simulink library "inp"  (R2021b)
settings: Solver=VariableStepAuto  StartTime=0.0  StopTime=10.0  RelTol=1e-3
undefined symbols (not defined in the file): C_TASK_5MS_S, FALSE, KINP_AcoreReadyToSlp_flg_ovrdflg, KINP_AcoreReadyToSlp_flg_ovrdval, KINP_AllowMovThd_OTA_enum_ovrdflg, KINP_AllowMovThd_OTA_enum_ovrdval, KINP_APSAngleTarget_Deg_ovrdflg, KINP_APSAngleTarget_Deg_ovrdval, KINP_APSDecReq_mps2_ovrdflg, KINP_APSDecReq_mps2_ovrdval, KINP_APSDecReqA_flg_ovrdflg, KINP_APSDecReqA_flg_ovrdval, KINP_APSDFLL_cm_ovrdflg, KINP_APSDFLL_cm_ovrdval, KINP_APSDFLR_cm_ovrdflg, KINP_APSDFLR_cm_ovrdval, KINP_APSDRLL_cm_ovrdflg, KINP_APSDRLL_cm_ovrdval, KINP_APSDRLR_cm_ovrdflg, KINP_APSDRLR_cm_ovrdval, KINP_APSExitCondition_enum_ovrdflg, KINP_APSExitCondition_enum_ovrdval, KINP_APSHWVer_enum_ovrdflg, KINP_APSHWVer_enum_ovrdval, KINP_APSProgressPCT_pct_ovrdflg, KINP_APSProgressPCT_pct_ovrdval, KINP_APSPwrReq_enum_ovrdflg, KINP_APSPwrReq_enum_ovrdval, KINP_APSReq_enum_ovrdflg, KINP_APSReq_enum_ovrdval, KINP_APSRQDisplay_enum_ovrdflg, KINP_APSRQDisplay_enum_ovrdval, KINP_APSRqEPASCtrl_flg_ovrdflg, KINP_APSRqEPASCtrl_flg_ovrdval, KINP_APSShiftPosnReq_enum_ovrdval, KINP_APSShiftPosnReq_enum_ovrflg, KINP_APSSpeedCMD_kph_ovrdval, KINP_APSSpeedCMD_kph_ovrflg, KINP_APSStaSystem_enum_ovrdflg, KINP_APSStaSystem_enum_ovrdval, KINP_APSSWVer_enum_ovrdflg, KINP_APSSWVer_enum_ovrdval, KINP_APSVMCReqA_flg_ovrdval, KINP_APSVMCReqA_flg_ovrflg, KINP_APSVRqEPASCtrl_flg_ovrdflg, KINP_APSVRqEPASCtrl_flg_ovrdval, KINP_AuxBattVolmV_mV_ovrdflg, KINP_AuxBattVolmV_mV_ovrdval, KINP_CAASSta_enum_ovrdflg, KINP_CAASSta_enum_ovrdval, KINP_CAASVMCReqA_flg_ovrdval, KINP_CAASVMCReqA_flg_ovrflg, KINP_CAN1BusOff_flg_ovrdflg, KINP_CAN1BusOff_flg_ovrdval, KINP_CAN2BusOff_flg_ovrdflg, KINP_CAN2BusOff_flg_ovrdval, KINP_CAN3BusOff_flg_ovrdflg, KINP_CAN3BusOff_flg_ovrdval, KINP_CAN4BusOff_flg_ovrdflg, KINP_CAN4BusOff_flg_ovrdval ... (+152)
libraries: FVT_lib x1035, hcu_lib x1
(part 18 of 33)

== system inp/INP/CAN3/SignalCheck/BMS1 ==
  BHAL_outputs : Inport
  inp_CanValid_bus : Inport  Port=2
  BMS1CSErr : FVT_lib/inp/can_signal_template  SystemSampleTime=-1  VariantActivationTime=update diagram  Latency=0  AutoFrameSizeCalculation=off
      link override defval: Value=KINP_BMS1CSErr_flg_defval
      link override ovrdflg: Value=KINP_BMS1CSErr_flg_ovrdflg
      link override ovrdval: Value=KINP_BMS1CSErr_flg_ovrdval
  BMS1RCErr : FVT_lib/inp/can_signal_template  SystemSampleTime=-1  VariantActivationTime=update diagram  Latency=0  AutoFrameSizeCalculation=off
      link override defval: Value=KINP_BMS1RCErr_flg_defval
      link override ovrdflg: Value=KINP_BMS1RCErr_flg_ovrdflg
      link override ovrdval: Value=KINP_BMS1RCErr_flg_ovrdval
  BMSChckSum1 : FVT_lib/inp/can_signal_template  SystemSampleTime=-1  VariantActivationTime=update diagram  Latency=0  AutoFrameSizeCalculation=off
      link override defval: Value=KINP_BMSChckSum1_enum_defval
      link override ovrdflg: Value=KINP_BMSChckSum1_enum_ovrdflg
      link override ovrdval: Value=KINP_BMSChckSum1_enum_ovrdval
  BMSRolCnct1 : FVT_lib/inp/can_signal_template  SystemSampleTime=-1  VariantActivationTime=update diagram  Latency=0  AutoFrameSizeCalculation=off
      link override defval: Value=KINP_BMSRolCnct1_enum_defval
      link override ovrdflg: Value=KINP_BMSRolCnct1_enum_ovrdflg
      link override ovrdval: Value=KINP_BMSRolCnct1_enum_ovrdval
  HVBPwrAvailChrg : FVT_lib/inp/can_signal_template  SystemSampleTime=-1  VariantActivationTime=update diagram  Latency=0  AutoFrameSizeCalculation=off
      link override defval: Value=KINP_HVBPwrAvailChrg_kW_defval
      link override ovrdflg: Value=KINP_HVBPwrAvailChrg_kW_ovrdflg
      link override ovrdval: Value=KINP_HVBPwrAvailChrg_kW_ovrdval
  HVBPwrAvailChrg30 : FVT_lib/inp/can_signal_template  SystemSampleTime=-1  VariantActivationTime=update diagram  Latency=0  AutoFrameSizeCalculation=off
      link override defval: Value=KINP_HVBPwrAvailChrg30_kW_defval
      link override ovrdflg: Value=KINP_HVBPwrAvailChrg30_kW_ovrdflg
      link override ovrdval: Value=KINP_HVBPwrAvailChrg30_kW_ovrdval
  HVBPwrAvailChrg60 : FVT_lib/inp/can_signal_template  SystemSampleTime=-1  VariantActivationTime=update diagram  Latency=0  AutoFrameSizeCalculation=off
      link override defval: Value=KINP_HVBPwrAvailChrg60_kW_defval
      link override ovrdflg: Value=KINP_HVBPwrAvailChrg60_kW_ovrdflg
      link override ovrdval: Value=KINP_HVBPwrAvailChrg60_kW_ovrdval
  HVBPwrAvailDchrg : FVT_lib/inp/can_signal_template  SystemSampleTime=-1  VariantActivationTime=update diagram  Latency=0  AutoFrameSizeCalculation=off
      link override defval: Value=KINP_HVBPwrAvailDchrg_kW_defval
      link override ovrdflg: Value=KINP_HVBPwrAvailDchrg_kW_ovrdflg
      link override ovrdval: Value=KINP_HVBPwrAvailDchrg_kW_ovrdval
  HVBPwrAvailDchrg30 : FVT_lib/inp/can_signal_template  SystemSampleTime=-1  VariantActivationTime=update diagram  Latency=0  AutoFrameSizeCalculation=off
      link override defval: Value=KINP_HVBPwrAvailDchrg30_kW_defval
      link override ovrdflg: Value=KINP_HVBPwrAvailDchrg30_kW_ovrdflg
      link override ovrdval: Value=KINP_HVBPwrAvailDchrg30_kW_ovrdval
  HVBPwrAvailDchrg60 : FVT_lib/inp/can_signal_template  SystemSampleTime=-1  VariantActivationTime=update diagram  Latency=0  AutoFrameSizeCalculation=off
      link override defval: Value=KINP_HVBPwrAvailDchrg60_kW_defval
      link override ovrdflg: Value=KINP_HVBPwrAvailDchrg60_kW_ovrdflg
      link override ovrdval: Value=KINP_HVBPwrAvailDchrg60_kW_ovrdval
  HVBattCurr : FVT_lib/inp/can_signal_template  SystemSampleTime=-1  VariantActivationTime=update diagram  Latency=0  AutoFrameSizeCalculation=off
      link override defval: Value=KINP_HVBattCurr_A_defval
      link override ovrdflg: Value=KINP_HVBattCurr_A_ovrdflg
      link override ovrdval: Value=KINP_HVBattCurr_A_ovrdval
  HVBattVolt : FVT_lib/inp/can_signal_template  SystemSampleTime=-1  VariantActivationTime=update diagram  Latency=0  AutoFrameSizeCalculation=off
      link override defval: Value=KINP_HVBattVolt_V_defval
      link override ovrdflg: Value=KINP_HVBattVolt_V_ovrdflg
      link override ovrdval: Value=KINP_HVBattVolt_V_ovrdval
  Terminator_{1..12} (12 alike) : Terminator
  True_VHAL_BMS1CSErr_flg : Constant  Value=TRUE  OutDataTypeStr=boolean
  True_VHAL_BMS1RCErr_flg : Constant  Value=TRUE  OutDataTypeStr=boolean
  True_VHAL_BMSChckSum1_enum : Constant  Value=TRUE  OutDataTypeStr=boolean
  True_VHAL_BMSRolCnct1_enum : Constant  Value=TRUE  OutDataTypeStr=boolean
  True_VHAL_HVBPwrAvailChrg30_kW : Constant  Value=TRUE  OutDataTypeStr=boolean
  True_VHAL_HVBPwrAvailChrg60_kW : Constant  Value=TRUE  OutDataTypeStr=boolean
  True_VHAL_HVBPwrAvailChrg_kW : Constant  Value=TRUE  OutDataTypeStr=boolean
  True_VHAL_HVBPwrAvailDchrg30_kW : Constant  Value=TRUE  OutDataTypeStr=boolean
  True_VHAL_HVBPwrAvailDchrg60_kW : Constant  Value=TRUE  OutDataTypeStr=boolean
  True_VHAL_HVBPwrAvailDchrg_kW : Constant  Value=TRUE  OutDataTypeStr=boolean
  True_VHAL_HVBattCurr_A : Constant  Value=TRUE  OutDataTypeStr=boolean
  True_VHAL_HVBattVolt_V : Constant  Value=TRUE  OutDataTypeStr=boolean
  slr1_{1..12} (12 alike) : BusSelector  OutputSignals=VINP_CANMsgValidBMS1_flg
  slr_VHAL_BMS1CSErr_flg : BusSelector  OutputSignals=VHAL_BMS1CSErr_flg
  slr_VHAL_BMS1RCErr_flg : BusSelector  OutputSignals=VHAL_BMS1RCErr_flg
  slr_VHAL_BMSChckSum1_enum : BusSelector  OutputSignals=VHAL_BMSChckSum1_enum
  slr_VHAL_BMSRolCnct1_enum : BusSelector  OutputSignals=VHAL_BMSRolCnct1_enum
  slr_VHAL_HVBPwrAvailChrg30_kW : BusSelector  OutputSignals=VHAL_HVBPwrAvailChrg30_kW
  slr_VHAL_HVBPwrAvailChrg60_kW : BusSelector  OutputSignals=VHAL_HVBPwrAvailChrg60_kW
  slr_VHAL_HVBPwrAvailChrg_kW : BusSelector  OutputSignals=VHAL_HVBPwrAvailChrg_kW
  slr_VHAL_HVBPwrAvailDchrg30_kW : BusSelector  OutputSignals=VHAL_HVBPwrAvailDchrg30_kW
  slr_VHAL_HVBPwrAvailDchrg60_kW : BusSelector  OutputSignals=VHAL_HVBPwrAvailDchrg60_kW
  slr_VHAL_HVBPwrAvailDchrg_kW : BusSelector  OutputSignals=VHAL_HVBPwrAvailDchrg_kW
  slr_VHAL_HVBattCurr_A : BusSelector  OutputSignals=VHAL_HVBattCurr_A
  slr_VHAL_HVBattVolt_V : BusSelector  OutputSignals=VHAL_HVBattVolt_V
  VINP_BMS1CSErr_flg : Outport
  VINP_BMS1RCErr_flg : Outport  Port=2
  VINP_BMSChckSum1_enum : Outport  Port=3
  VINP_BMSRolCnct1_enum : Outport  Port=4
  VINP_HVBPwrAvailChrg_kW : Outport  Port=5
  VINP_HVBPwrAvailChrg30_kW : Outport  Port=6
  VINP_HVBPwrAvailChrg60_kW : Outport  Port=7
  VINP_HVBPwrAvailDchrg_kW : Outport  Port=8
  VINP_HVBPwrAvailDchrg30_kW : Outport  Port=9
  VINP_HVBPwrAvailDchrg60_kW : Outport  Port=10
  VINP_HVBattCurr_A : Outport  Port=11
  VINP_HVBattVolt_V : Outport  Port=12
  wires:
  BHAL_outputs/1 -> [BHAL_outputs]
  inp_CanValid_bus/1 -> [inp_CanValid_bus]
  [BHAL_outputs] -> slr_VHAL_BMS1CSErr_flg/1
  slr_VHAL_BMS1CSErr_flg/1 -> BMS1CSErr/1  "<VHAL_BMS1CSErr_flg>"
  True_VHAL_BMS1CSErr_flg/1 -> BMS1CSErr/2
  [inp_CanValid_bus] -> slr1_1/1
  slr1_1/1 -> BMS1CSErr/3  "<VINP_CANMsgValidBMS1_flg>"
  BMS1CSErr/1 -> VINP_BMS1CSErr_flg/1  "VINP_BMS1CSErr_flg"
  BMS1CSErr/2 -> Terminator_1/1
  [BHAL_outputs] -> slr_VHAL_BMS1RCErr_flg/1
  slr_VHAL_BMS1RCErr_flg/1 -> BMS1RCErr/1  "<VHAL_BMS1RCErr_flg>"
  True_VHAL_BMS1RCErr_flg/1 -> BMS1RCErr/2
  [inp_CanValid_bus] -> slr1_2/1
  slr1_2/1 -> BMS1RCErr/3  "<VINP_CANMsgValidBMS1_flg>"
  BMS1RCErr/1 -> VINP_BMS1RCErr_flg/1  "VINP_BMS1RCErr_flg"
  BMS1RCErr/2 -> Terminator_2/1
  [BHAL_outputs] -> slr_VHAL_BMSChckSum1_enum/1
  slr_VHAL_BMSChckSum1_enum/1 -> BMSChckSum1/1  "<VHAL_BMSChckSum1_enum>"
  True_VHAL_BMSChckSum1_enum/1 -> BMSChckSum1/2
  [inp_CanValid_bus] -> slr1_3/1
  slr1_3/1 -> BMSChckSum1/3  "<VINP_CANMsgValidBMS1_flg>"
  BMSChckSum1/1 -> VINP_BMSChckSum1_enum/1  "VINP_BMSChckSum1_enum"
  BMSChckSum1/2 -> Terminator_3/1
  [BHAL_outputs] -> slr_VHAL_BMSRolCnct1_enum/1
  slr_VHAL_BMSRolCnct1_enum/1 -> BMSRolCnct1/1  "<VHAL_BMSRolCnct1_enum>"
  True_VHAL_BMSRolCnct1_enum/1 -> BMSRolCnct1/2
  [inp_CanValid_bus] -> slr1_4/1
  slr1_4/1 -> BMSRolCnct1/3  "<VINP_CANMsgValidBMS1_flg>"
  BMSRolCnct1/1 -> VINP_BMSRolCnct1_enum/1  "VINP_BMSRolCnct1_enum"
  BMSRolCnct1/2 -> Terminator_4/1
  [BHAL_outputs] -> slr_VHAL_HVBPwrAvailChrg_kW/1
  slr_VHAL_HVBPwrAvailChrg_kW/1 -> HVBPwrAvailChrg/1  "<VHAL_HVBPwrAvailChrg_kW>"
  True_VHAL_HVBPwrAvailChrg_kW/1 -> HVBPwrAvailChrg/2
  [inp_CanValid_bus] -> slr1_5/1
  slr1_5/1 -> HVBPwrAvailChrg/3  "<VINP_CANMsgValidBMS1_flg>"
  HVBPwrAvailChrg/1 -> VINP_HVBPwrAvailChrg_kW/1  "VINP_HVBPwrAvailChrg_kW"
  HVBPwrAvailChrg/2 -> Terminator_5/1
  [BHAL_outputs] -> slr_VHAL_HVBPwrAvailChrg30_kW/1
  slr_VHAL_HVBPwrAvailChrg30_kW/1 -> HVBPwrAvailChrg30/1  "<VHAL_HVBPwrAvailChrg30_kW>"
  True_VHAL_HVBPwrAvailChrg30_kW/1 -> HVBPwrAvailChrg30/2
  [inp_CanValid_bus] -> slr1_6/1
  slr1_6/1 -> HVBPwrAvailChrg30/3  "<VINP_CANMsgValidBMS1_flg>"
  HVBPwrAvailChrg30/1 -> VINP_HVBPwrAvailChrg30_kW/1  "VINP_HVBPwrAvailChrg30_kW"
  HVBPwrAvailChrg30/2 -> Terminator_6/1
  [BHAL_outputs] -> slr_VHAL_HVBPwrAvailChrg60_kW/1
  slr_VHAL_HVBPwrAvailChrg60_kW/1 -> HVBPwrAvailChrg60/1  "<VHAL_HVBPwrAvailChrg60_kW>"
  True_VHAL_HVBPwrAvailChrg60_kW/1 -> HVBPwrAvailChrg60/2
  [inp_CanValid_bus] -> slr1_7/1
  slr1_7/1 -> HVBPwrAvailChrg60/3  "<VINP_CANMsgValidBMS1_flg>"
  HVBPwrAvailChrg60/1 -> VINP_HVBPwrAvailChrg60_kW/1  "VINP_HVBPwrAvailChrg60_kW"
  HVBPwrAvailChrg60/2 -> Terminator_7/1
  [BHAL_outputs] -> slr_VHAL_HVBPwrAvailDchrg_kW/1
  slr_VHAL_HVBPwrAvailDchrg_kW/1 -> HVBPwrAvailDchrg/1  "<VHAL_HVBPwrAvailDchrg_kW>"
  True_VHAL_HVBPwrAvailDchrg_kW/1 -> HVBPwrAvailDchrg/2
  [inp_CanValid_bus] -> slr1_8/1
  slr1_8/1 -> HVBPwrAvailDchrg/3  "<VINP_CANMsgValidBMS1_flg>"
  HVBPwrAvailDchrg/1 -> VINP_HVBPwrAvailDchrg_kW/1  "VINP_HVBPwrAvailDchrg_kW"
  HVBPwrAvailDchrg/2 -> Terminator_8/1
  [BHAL_outputs] -> slr_VHAL_HVBPwrAvailDchrg30_kW/1
  slr_VHAL_HVBPwrAvailDchrg30_kW/1 -> HVBPwrAvailDchrg30/1  "<VHAL_HVBPwrAvailDchrg30_kW>"
  True_VHAL_HVBPwrAvailDchrg30_kW/1 -> HVBPwrAvailDchrg30/2
  [inp_CanValid_bus] -> slr1_9/1
  slr1_9/1 -> HVBPwrAvailDchrg30/3  "<VINP_CANMsgValidBMS1_flg>"
  HVBPwrAvailDchrg30/1 -> VINP_HVBPwrAvailDchrg30_kW/1  "VINP_HVBPwrAvailDchrg30_kW"
  HVBPwrAvailDchrg30/2 -> Terminator_9/1
  [BHAL_outputs] -> slr_VHAL_HVBPwrAvailDchrg60_kW/1
  slr_VHAL_HVBPwrAvailDchrg60_kW/1 -> HVBPwrAvailDchrg60/1  "<VHAL_HVBPwrAvailDchrg60_kW>"
  True_VHAL_HVBPwrAvailDchrg60_kW/1 -> HVBPwrAvailDchrg60/2
  [inp_CanValid_bus] -> slr1_10/1
  slr1_10/1 -> HVBPwrAvailDchrg60/3  "<VINP_CANMsgValidBMS1_flg>"
  HVBPwrAvailDchrg60/1 -> VINP_HVBPwrAvailDchrg60_kW/1  "VINP_HVBPwrAvailDchrg60_kW"
  HVBPwrAvailDchrg60/2 -> Terminator_10/1
  [BHAL_outputs] -> slr_VHAL_HVBattCurr_A/1
  slr_VHAL_HVBattCurr_A/1 -> HVBattCurr/1  "<VHAL_HVBattCurr_A>"
  True_VHAL_HVBattCurr_A/1 -> HVBattCurr/2
  [inp_CanValid_bus] -> slr1_11/1
  slr1_11/1 -> HVBattCurr/3  "<VINP_CANMsgValidBMS1_flg>"
  HVBattCurr/1 -> VINP_HVBattCurr_A/1  "VINP_HVBattCurr_A"
  HVBattCurr/2 -> Terminator_11/1
  [BHAL_outputs] -> slr_VHAL_HVBattVolt_V/1
  slr_VHAL_HVBattVolt_V/1 -> HVBattVolt/1  "<VHAL_HVBattVolt_V>"
  True_VHAL_HVBattVolt_V/1 -> HVBattVolt/2
  [inp_CanValid_bus] -> slr1_12/1
  slr1_12/1 -> HVBattVolt/3  "<VINP_CANMsgValidBMS1_flg>"
  HVBattVolt/1 -> VINP_HVBattVolt_V/1  "VINP_HVBattVolt_V"
  HVBattVolt/2 -> Terminator_12/1

== system inp/INP/CAN3/SignalCheck/BMS3 ==
  BHAL_outputs : Inport
  inp_CanValid_bus : Inport  Port=2
  ACChrgCurrDis : FVT_lib/inp/can_signal_template  SystemSampleTime=-1  VariantActivationTime=update diagram  Latency=0  AutoFrameSizeCalculation=off
      link override defval: Value=KINP_ACChrgCurrDis_A_defval
      link override ovrdflg: Value=KINP_ACChrgCurrDis_A_ovrdflg
      link override ovrdval: Value=KINP_ACChrgCurrDis_A_ovrdval
  FireDetErr : FVT_lib/inp/can_signal_template  SystemSampleTime=-1  VariantActivationTime=update diagram  Latency=0  AutoFrameSizeCalculation=off
      link override defval: Value=KINP_FireDetErr_flg_defval
      link override ovrdflg: Value=KINP_FireDetErr_flg_ovrdflg
      link override ovrdval: Value=KINP_FireDetErr_flg_ovrdval
  HVBChrgPwr : FVT_lib/inp/can_signal_template  SystemSampleTime=-1  VariantActivationTime=update diagram  Latency=0  AutoFrameSizeCalculation=off
      link override defval: Value=KINP_HVBChrgPwr_kWh_defval
      link override ovrdflg: Value=KINP_HVBChrgPwr_kWh_ovrdflg
      link override ovrdval: Value=KINP_HVBChrgPwr_kWh_ovrdval
  HVBChrgPwrTotal : FVT_lib/inp/can_signal_template  SystemSampleTime=-1  VariantActivationTime=update diagram  Latency=0  AutoFrameSizeCalculation=off
      link override defval: Value=KINP_HVBChrgPwrTotal_kWh_defval
      link override ovrdflg: Value=KINP_HVBChrgPwrTotal_kWh_ovrdflg
      link override ovrdval: Value=KINP_HVBChrgPwrTotal_kWh_ovrdval
  HVBDrvPwr : FVT_lib/inp/can_signal_template  SystemSampleTime=-1  VariantActivationTime=update diagram  Latency=0  AutoFrameSizeCalculation=off
      link override defval: Value=KINP_HVBDrvPwr_kWh_defval
      link override ovrdflg: Value=KINP_HVBDrvPwr_kWh_ovrdflg
      link override ovrdval: Value=KINP_HVBDrvPwr_kWh_ovrdval
  HVBDrvPwrTotal : FVT_lib/inp/can_signal_template  SystemSampleTime=-1  VariantActivationTime=update diagram  Latency=0  AutoFrameSizeCalculation=off
      link override defval: Value=KINP_HVBDrvPwrTotal_kWh_defval
      link override ovrdflg: Value=KINP_HVBDrvPwrTotal_kWh_ovrdflg
      link override ovrdval: Value=KINP_HVBDrvPwrTotal_kWh_ovrdval
  HVBFullChrgPwr : FVT_lib/inp/can_signal_template  SystemSampleTime=-1  VariantActivationTime=update diagram  Latency=0  AutoFrameSizeCalculation=off
      link override defval: Value=KINP_HVBFullChrgPwr_kWh_defval
      link override ovrdflg: Value=KINP_HVBFullChrgPwr_kWh_ovrdflg
      link override ovrdval: Value=KINP_HVBFullChrgPwr_kWh_ovrdval
  HVBIsoImpedenceN : FVT_lib/inp/can_signal_template  SystemSampleTime=-1  VariantActivationTime=update diagram  Latency=0  AutoFrameSizeCalculation=off
      link override defval: Value=KINP_HVBIsoImpedenceN_Megaohm_defval
      link override ovrdflg: Value=KINP_HVBIsoImpedenceN_Megaohm_ovrdflg
      link override ovrdval: Value=KINP_HVBIsoImpedenceN_Megaohm_ovrdval
  HVBIsoImpedenceP : FVT_lib/inp/can_signal_template  SystemSampleTime=-1  VariantActivationTime=update diagram  Latency=0  AutoFrameSizeCalculation=off
      link override defval: Value=KINP_HVBIsoImpedenceP_Megaohm_defval
      link override ovrdflg: Value=KINP_HVBIsoImpedenceP_Megaohm_ovrdflg
      link override ovrdval: Value=KINP_HVBIsoImpedenceP_Megaohm_ovrdval
  HVBSOH : FVT_lib/inp/can_signal_template  SystemSampleTime=-1  VariantActivationTime=update diagram  Latency=0  AutoFrameSizeCalculation=off
      link override defval: Value=KINP_HVBSOH_pct_defval
      link override ovrdflg: Value=KINP_HVBSOH_pct_ovrdflg
      link override ovrdval: Value=KINP_HVBSOH_pct_ovrdval
  HVBattErr : FVT_lib/inp/can_signal_template  SystemSampleTime=-1  VariantActivationTime=update diagram  Latency=0  AutoFrameSizeCalculation=off
      link override defval: Value=KINP_HVBattErr_flg_defval
      link override ovrdflg: Value=KINP_HVBattErr_flg_ovrdflg
      link override ovrdval: Value=KINP_HVBattErr_flg_ovrdval
  HVBattPackVolt : FVT_lib/inp/can_signal_template  SystemSampleTime=-1  VariantActivationTime=update diagram  Latency=0  AutoFrameSizeCalculation=off
      link override defval: Value=KINP_HVBattPackVolt_V_defval
      link override ovrdflg: Value=KINP_HVBattPackVolt_V_ovrdflg
      link override ovrdval: Value=KINP_HVBattPackVolt_V_ovrdval
  HVBattSOC : FVT_lib/inp/can_signal_template  SystemSampleTime=-1  VariantActivationTime=update diagram  Latency=0  AutoFrameSizeCalculation=off
      link override defval: Value=KINP_HVBattSOC_pct_defval
      link override ovrdflg: Value=KINP_HVBattSOC_pct_ovrdflg
      link override ovrdval: Value=KINP_HVBattSOC_pct_ovrdval
  HVBattSOCDis : FVT_lib/inp/can_signal_template  SystemSampleTime=-1  VariantActivationTime=update diagram  Latency=0  AutoFrameSizeCalculation=off
      link override defval: Value=KINP_HVBattSOCDis_pct_defval
      link override ovrdflg: Value=KINP_HVBattSOCDis_pct_ovrdflg
      link override ovrdval: Value=KINP_HVBattSOCDis_pct_ovrdval
  RemainChrgTime : FVT_lib/inp/can_signal_template  SystemSampleTime=-1  VariantActivationTime=update diagram  Latency=0  AutoFrameSizeCalculation=off
      link override defval: Value=KINP_RemainChrgTime_min_defval
      link override ovrdflg: Value=KINP_RemainChrgTime_min_ovrdflg
      link override ovrdval: Value=KINP_RemainChrgTime_min_ovrdval
  Terminator_{1..15} (15 alike) : Terminator
  True_VHAL_ACChrgCurrDis_A : Constant  Value=TRUE  OutDataTypeStr=boolean
  True_VHAL_FireDetErr_flg : Constant  Value=TRUE  OutDataTypeStr=boolean
  True_VHAL_HVBChrgPwrTotal_kWh : Constant  Value=TRUE  OutDataTypeStr=boolean
  True_VHAL_HVBChrgPwr_kWh : Constant  Value=TRUE  OutDataTypeStr=boolean
  True_VHAL_HVBDrvPwrTotal_kWh : Constant  Value=TRUE  OutDataTypeStr=boolean
  True_VHAL_HVBDrvPwr_kWh : Constant  Value=TRUE  OutDataTypeStr=boolean
  True_VHAL_HVBFullChrgPwr_kWh : Constant  Value=TRUE  OutDataTypeStr=boolean
  True_VHAL_HVBIsoImpedenceN_Megaohm : Constant  Value=TRUE  OutDataTypeStr=boolean
  True_VHAL_HVBIsoImpedenceP_Megaohm : Constant  Value=TRUE  OutDataTypeStr=boolean
  True_VHAL_HVBSOH_pct : Constant  Value=TRUE  OutDataTypeStr=boolean
  True_VHAL_HVBattErr_flg : Constant  Value=TRUE  OutDataTypeStr=boolean
  True_VHAL_HVBattPackVolt_V : Constant  Value=TRUE  OutDataTypeStr=boolean
  True_VHAL_HVBattSOCDis_pct : Constant  Value=TRUE  OutDataTypeStr=boolean
  True_VHAL_HVBattSOC_pct : Constant  Value=TRUE  OutDataTypeStr=boolean
  True_VHAL_RemainChrgTime_min : Constant  Value=TRUE  OutDataTypeStr=boolean
  slr1_{1..15} (15 alike) : BusSelector  OutputSignals=VINP_CANMsgValidBMS3_flg
  slr_VHAL_ACChrgCurrDis_A : BusSelector  OutputSignals=VHAL_ACChrgCurrDis_A
  slr_VHAL_FireDetErr_flg : BusSelector  OutputSignals=VHAL_FireDetErr_flg
  slr_VHAL_HVBChrgPwrTotal_kWh : BusSelector  OutputSignals=VHAL_HVBChrgPwrTotal_kWh
  slr_VHAL_HVBChrgPwr_kWh : BusSelector  OutputSignals=VHAL_HVBChrgPwr_kWh
  slr_VHAL_HVBDrvPwrTotal_kWh : BusSelector  OutputSignals=VHAL_HVBDrvPwrTotal_kWh
  slr_VHAL_HVBDrvPwr_kWh : BusSelector  OutputSignals=VHAL_HVBDrvPwr_kWh
  slr_VHAL_HVBFullChrgPwr_kWh : BusSelector  OutputSignals=VHAL_HVBFullChrgPwr_kWh
  slr_VHAL_HVBIsoImpedenceN_Megaohm : BusSelector  OutputSignals=VHAL_HVBIsoImpedenceN_Megaohm
  slr_VHAL_HVBIsoImpedenceP_Megaohm : BusSelector  OutputSignals=VHAL_HVBIsoImpedenceP_Megaohm
  slr_VHAL_HVBSOH_pct : BusSelector  OutputSignals=VHAL_HVBSOH_pct
  slr_VHAL_HVBattErr_flg : BusSelector  OutputSignals=VHAL_HVBattErr_flg
  slr_VHAL_HVBattPackVolt_V : BusSelector  OutputSignals=VHAL_HVBattPackVolt_V
  slr_VHAL_HVBattSOCDis_pct : BusSelector  OutputSignals=VHAL_HVBattSOCDis_pct
  slr_VHAL_HVBattSOC_pct : BusSelector  OutputSignals=VHAL_HVBattSOC_pct
  slr_VHAL_RemainChrgTime_min : BusSelector  OutputSignals=VHAL_RemainChrgTime_min
  VINP_ACChrgCurrDis_A : Outport
  VINP_FireDetErr_flg : Outport  Port=2
  VINP_HVBChrgPwr_kWh : Outport  Port=3
  VINP_HVBChrgPwrTotal_kWh : Outport  Port=4
  VINP_HVBDrvPwr_kWh : Outport  Port=5
  VINP_HVBDrvPwrTotal_kWh : Outport  Port=6
  VINP_HVBFullChrgPwr_kWh : Outport  Port=7
  VINP_HVBIsoImpedenceN_Megaohm : Outport  Port=8
  VINP_HVBIsoImpedenceP_Megaohm : Outport  Port=9
  VINP_HVBSOH_pct : Outport  Port=10
  VINP_HVBattErr_flg : Outport  Port=11
  VINP_HVBattPackVolt_V : Outport  Port=12
  VINP_HVBattSOC_pct : Outport  Port=13
  VINP_HVBattSOCDis_pct : Outport  Port=14
  VINP_RemainChrgTime_min : Outport  Port=15
  wires:
  BHAL_outputs/1 -> [BHAL_outputs]
  inp_CanValid_bus/1 -> [inp_CanValid_bus]
  [BHAL_outputs] -> slr_VHAL_ACChrgCurrDis_A/1
  slr_VHAL_ACChrgCurrDis_A/1 -> ACChrgCurrDis/1  "<VHAL_ACChrgCurrDis_A>"
  True_VHAL_ACChrgCurrDis_A/1 -> ACChrgCurrDis/2
  [inp_CanValid_bus] -> slr1_1/1
  slr1_1/1 -> ACChrgCurrDis/3  "<VINP_CANMsgValidBMS3_flg>"
  ACChrgCurrDis/1 -> VINP_ACChrgCurrDis_A/1  "VINP_ACChrgCurrDis_A"
  ACChrgCurrDis/2 -> Terminator_1/1
  [BHAL_outputs] -> slr_VHAL_FireDetErr_flg/1
  slr_VHAL_FireDetErr_flg/1 -> FireDetErr/1  "<VHAL_FireDetErr_flg>"
  True_VHAL_FireDetErr_flg/1 -> FireDetErr/2
  [inp_CanValid_bus] -> slr1_2/1
  slr1_2/1 -> FireDetErr/3  "<VINP_CANMsgValidBMS3_flg>"
  FireDetErr/1 -> VINP_FireDetErr_flg/1  "VINP_FireDetErr_flg"
  FireDetErr/2 -> Terminator_2/1
  [BHAL_outputs] -> slr_VHAL_HVBChrgPwr_kWh/1
  slr_VHAL_HVBChrgPwr_kWh/1 -> HVBChrgPwr/1  "<VHAL_HVBChrgPwr_kWh>"
  True_VHAL_HVBChrgPwr_kWh/1 -> HVBChrgPwr/2
  [inp_CanValid_bus] -> slr1_3/1
  slr1_3/1 -> HVBChrgPwr/3  "<VINP_CANMsgValidBMS3_flg>"
  HVBChrgPwr/1 -> VINP_HVBChrgPwr_kWh/1  "VINP_HVBChrgPwr_kWh"
  HVBChrgPwr/2 -> Terminator_3/1
  [BHAL_outputs] -> slr_VHAL_HVBChrgPwrTotal_kWh/1
  slr_VHAL_HVBChrgPwrTotal_kWh/1 -> HVBChrgPwrTotal/1  "<VHAL_HVBChrgPwrTotal_kWh>"
  True_VHAL_HVBChrgPwrTotal_kWh/1 -> HVBChrgPwrTotal/2
  [inp_CanValid_bus] -> slr1_4/1
  slr1_4/1 -> HVBChrgPwrTotal/3  "<VINP_CANMsgValidBMS3_flg>"
  HVBChrgPwrTotal/1 -> VINP_HVBChrgPwrTotal_kWh/1  "VINP_HVBChrgPwrTotal_kWh"
  HVBChrgPwrTotal/2 -> Terminator_4/1
  [BHAL_outputs] -> slr_VHAL_HVBDrvPwr_kWh/1
  slr_VHAL_HVBDrvPwr_kWh/1 -> HVBDrvPwr/1  "<VHAL_HVBDrvPwr_kWh>"
  True_VHAL_HVBDrvPwr_kWh/1 -> HVBDrvPwr/2
  [inp_CanValid_bus] -> slr1_5/1
  slr1_5/1 -> HVBDrvPwr/3  "<VINP_CANMsgValidBMS3_flg>"
  HVBDrvPwr/1 -> VINP_HVBDrvPwr_kWh/1  "VINP_HVBDrvPwr_kWh"
  HVBDrvPwr/2 -> Terminator_5/1
  [BHAL_outputs] -> slr_VHAL_HVBDrvPwrTotal_kWh/1
  slr_VHAL_HVBDrvPwrTotal_kWh/1 -> HVBDrvPwrTotal/1  "<VHAL_HVBDrvPwrTotal_kWh>"
  True_VHAL_HVBDrvPwrTotal_kWh/1 -> HVBDrvPwrTotal/2
  [inp_CanValid_bus] -> slr1_6/1
  slr1_6/1 -> HVBDrvPwrTotal/3  "<VINP_CANMsgValidBMS3_flg>"
  HVBDrvPwrTotal/1 -> VINP_HVBDrvPwrTotal_kWh/1  "VINP_HVBDrvPwrTotal_kWh"
  HVBDrvPwrTotal/2 -> Terminator_6/1
  [BHAL_outputs] -> slr_VHAL_HVBFullChrgPwr_kWh/1
  slr_VHAL_HVBFullChrgPwr_kWh/1 -> HVBFullChrgPwr/1  "<VHAL_HVBFullChrgPwr_kWh>"
  True_VHAL_HVBFullChrgPwr_kWh/1 -> HVBFullChrgPwr/2
  [inp_CanValid_bus] -> slr1_7/1
  slr1_7/1 -> HVBFullChrgPwr/3  "<VINP_CANMsgValidBMS3_flg>"
  HVBFullChrgPwr/1 -> VINP_HVBFullChrgPwr_kWh/1  "VINP_HVBFullChrgPwr_kWh"
  HVBFullChrgPwr/2 -> Terminator_7/1
  [BHAL_outputs] -> slr_VHAL_HVBIsoImpedenceN_Megaohm/1
  slr_VHAL_HVBIsoImpedenceN_Megaohm/1 -> HVBIsoImpedenceN/1  "<VHAL_HVBIsoImpedenceN_Megaohm>"
  True_VHAL_HVBIsoImpedenceN_Megaohm/1 -> HVBIsoImpedenceN/2
  [inp_CanValid_bus] -> slr1_8/1
  slr1_8/1 -> HVBIsoImpedenceN/3  "<VINP_CANMsgValidBMS3_flg>"
  HVBIsoImpedenceN/1 -> VINP_HVBIsoImpedenceN_Megaohm/1  "VINP_HVBIsoImpedenceN_Megaohm"
  HVBIsoImpedenceN/2 -> Terminator_8/1
  [BHAL_outputs] -> slr_VHAL_HVBIsoImpedenceP_Megaohm/1
  slr_VHAL_HVBIsoImpedenceP_Megaohm/1 -> HVBIsoImpedenceP/1  "<VHAL_HVBIsoImpedenceP_Megaohm>"
  True_VHAL_HVBIsoImpedenceP_Megaohm/1 -> HVBIsoImpedenceP/2
  [inp_CanValid_bus] -> slr1_9/1
  slr1_9/1 -> HVBIsoImpedenceP/3  "<VINP_CANMsgValidBMS3_flg>"
  HVBIsoImpedenceP/1 -> VINP_HVBIsoImpedenceP_Megaohm/1  "VINP_HVBIsoImpedenceP_Megaohm"
  HVBIsoImpedenceP/2 -> Terminator_9/1
  [BHAL_outputs] -> slr_VHAL_HVBSOH_pct/1
  slr_VHAL_HVBSOH_pct/1 -> HVBSOH/1  "<VHAL_HVBSOH_pct>"
  True_VHAL_HVBSOH_pct/1 -> HVBSOH/2
  [inp_CanValid_bus] -> slr1_10/1
  slr1_10/1 -> HVBSOH/3  "<VINP_CANMsgValidBMS3_flg>"
  HVBSOH/1 -> VINP_HVBSOH_pct/1  "VINP_HVBSOH_pct"
  HVBSOH/2 -> Terminator_10/1
  [BHAL_outputs] -> slr_VHAL_HVBattErr_flg/1
  slr_VHAL_HVBattErr_flg/1 -> HVBattErr/1  "<VHAL_HVBattErr_flg>"
  True_VHAL_HVBattErr_flg/1 -> HVBattErr/2
  [inp_CanValid_bus] -> slr1_11/1
  slr1_11/1 -> HVBattErr/3  "<VINP_CANMsgValidBMS3_flg>"
  HVBattErr/1 -> VINP_HVBattErr_flg/1  "VINP_HVBattErr_flg"
  HVBattErr/2 -> Terminator_11/1
  [BHAL_outputs] -> slr_VHAL_HVBattPackVolt_V/1
  slr_VHAL_HVBattPackVolt_V/1 -> HVBattPackVolt/1  "<VHAL_HVBattPackVolt_V>"
  True_VHAL_HVBattPackVolt_V/1 -> HVBattPackVolt/2
  [inp_CanValid_bus] -> slr1_12/1
  slr1_12/1 -> HVBattPackVolt/3  "<VINP_CANMsgValidBMS3_flg>"
  HVBattPackVolt/1 -> VINP_HVBattPackVolt_V/1  "VINP_HVBattPackVolt_V"
  HVBattPackVolt/2 -> Terminator_12/1
  [BHAL_outputs] -> slr_VHAL_HVBattSOC_pct/1
  slr_VHAL_HVBattSOC_pct/1 -> HVBattSOC/1  "<VHAL_HVBattSOC_pct>"
  True_VHAL_HVBattSOC_pct/1 -> HVBattSOC/2
  [inp_CanValid_bus] -> slr1_13/1
  slr1_13/1 -> HVBattSOC/3  "<VINP_CANMsgValidBMS3_flg>"
  HVBattSOC/1 -> VINP_HVBattSOC_pct/1  "VINP_HVBattSOC_pct"
  HVBattSOC/2 -> Terminator_13/1
  [BHAL_outputs] -> slr_VHAL_HVBattSOCDis_pct/1
  slr_VHAL_HVBattSOCDis_pct/1 -> HVBattSOCDis/1  "<VHAL_HVBattSOCDis_pct>"
  True_VHAL_HVBattSOCDis_pct/1 -> HVBattSOCDis/2
  [inp_CanValid_bus] -> slr1_14/1
  slr1_14/1 -> HVBattSOCDis/3  "<VINP_CANMsgValidBMS3_flg>"
  HVBattSOCDis/1 -> VINP_HVBattSOCDis_pct/1  "VINP_HVBattSOCDis_pct"
  HVBattSOCDis/2 -> Terminator_14/1
  [BHAL_outputs] -> slr_VHAL_RemainChrgTime_min/1
  slr_VHAL_RemainChrgTime_min/1 -> RemainChrgTime/1  "<VHAL_RemainChrgTime_min>"
  True_VHAL_RemainChrgTime_min/1 -> RemainChrgTime/2
  [inp_CanValid_bus] -> slr1_15/1
  slr1_15/1 -> RemainChrgTime/3  "<VINP_CANMsgValidBMS3_flg>"
  RemainChrgTime/1 -> VINP_RemainChrgTime_min/1  "VINP_RemainChrgTime_min"
  RemainChrgTime/2 -> Terminator_15/1

== system inp/INP/CAN3/SignalCheck/BMS4 ==
  BHAL_outputs : Inport
  inp_CanValid_bus : Inport  Port=2
  CellTempAvg : FVT_lib/inp/can_signal_template  SystemSampleTime=-1  VariantActivationTime=update diagram  Latency=0  AutoFrameSizeCalculation=off
      link override defval: Value=KINP_CellTempAvg_C_defval
      link override ovrdflg: Value=KINP_CellTempAvg_C_ovrdflg
      link override ovrdval: Value=KINP_CellTempAvg_C_ovrdval
  HVBCellVoltMax : FVT_lib/inp/can_signal_template  SystemSampleTime=-1  VariantActivationTime=update diagram  Latency=0  AutoFrameSizeCalculation=off
      link override defval: Value=KINP_HVBCellVoltMax_mV_defval
      link override ovrdflg: Value=KINP_HVBCellVoltMax_mV_ovrdflg
      link override ovrdval: Value=KINP_HVBCellVoltMax_mV_ovrdval
  HVBCellVoltMin : FVT_lib/inp/can_signal_template  SystemSampleTime=-1  VariantActivationTime=update diagram  Latency=0  AutoFrameSizeCalculation=off
      link override defval: Value=KINP_HVBCellVoltMin_mV_defval
      link override ovrdflg: Value=KINP_HVBCellVoltMin_mV_ovrdflg
      link override ovrdval: Value=KINP_HVBCellVoltMin_mV_ovrdval
  HVBMTempMax : FVT_lib/inp/can_signal_template  SystemSampleTime=-1  VariantActivationTime=update diagram  Latency=0  AutoFrameSizeCalculation=off
      link override defval: Value=KINP_HVBMTempMax_C_defval
      link override ovrdflg: Value=KINP_HVBMTempMax_C_ovrdflg
      link override ovrdval: Value=KINP_HVBMTempMax_C_ovrdval
  HVBMTempMin : FVT_lib/inp/can_signal_template  SystemSampleTime=-1  VariantActivationTime=update diagram  Latency=0  AutoFrameSizeCalculation=off
      link override defval: Value=KINP_HVBMTempMin_C_defval
      link override ovrdflg: Value=KINP_HVBMTempMin_C_ovrdflg
      link override ovrdval: Value=KINP_HVBMTempMin_C_ovrdval
  MaxCellTempNum : FVT_lib/inp/can_signal_template  SystemSampleTime=-1  VariantActivationTime=update diagram  Latency=0  AutoFrameSizeCalculation=off
      link override defval: Value=KINP_MaxCellTempNum_enum_defval
      link override ovrdflg: Value=KINP_MaxCellTempNum_enum_ovrdflg
      link override ovrdval: Value=KINP_MaxCellTempNum_enum_ovrdval
  MaxCellVoltNum : FVT_lib/inp/can_signal_template  SystemSampleTime=-1  VariantActivationTime=update diagram  Latency=0  AutoFrameSizeCalculation=off
      link override defval: Value=KINP_MaxCellVoltNum_enum_defval
      link override ovrdflg: Value=KINP_MaxCellVoltNum_enum_ovrdflg
      link override ovrdval: Value=KINP_MaxCellVoltNum_enum_ovrdval
  MinCellTempNum : FVT_lib/inp/can_signal_template  SystemSampleTime=-1  VariantActivationTime=update diagram  Latency=0  AutoFrameSizeCalculation=off
      link override defval: Value=KINP_MinCellTempNum_enum_defval
      link override ovrdflg: Value=KINP_MinCellTempNum_enum_ovrdflg
      link override ovrdval: Value=KINP_MinCellTempNum_enum_ovrdval
  MinCellVoltNum : FVT_lib/inp/can_signal_template  SystemSampleTime=-1  VariantActivationTime=update diagram  Latency=0  AutoFrameSizeCalculation=off
      link override defval: Value=KINP_MinCellVoltNum_enum_defval
      link override ovrdflg: Value=KINP_MinCellVoltNum_enum_ovrdflg
      link override ovrdval: Value=KINP_MinCellVoltNum_enum_ovrdval
  Terminator_{1..9} (9 alike) : Terminator
  True_VHAL_CellTempAvg_C : Constant  Value=TRUE  OutDataTypeStr=boolean
  True_VHAL_HVBCellVoltMax_mV : Constant  Value=TRUE  OutDataTypeStr=boolean
  True_VHAL_HVBCellVoltMin_mV : Constant  Value=TRUE  OutDataTypeStr=boolean
  True_VHAL_HVBMTempMax_C : Constant  Value=TRUE  OutDataTypeStr=boolean
  True_VHAL_HVBMTempMin_C : Constant  Value=TRUE  OutDataTypeStr=boolean
  True_VHAL_MaxCellTempNum_enum : Constant  Value=TRUE  OutDataTypeStr=boolean
  True_VHAL_MaxCellVoltNum_enum : Constant  Value=TRUE  OutDataTypeStr=boolean
  True_VHAL_MinCellTempNum_enum : Constant  Value=TRUE  OutDataTypeStr=boolean
  True_VHAL_MinCellVoltNum_enum : Constant  Value=TRUE  OutDataTypeStr=boolean
  slr1_{1..9} (9 alike) : BusSelector  OutputSignals=VINP_CANMsgValidBMS4_flg
  slr_VHAL_CellTempAvg_C : BusSelector  OutputSignals=VHAL_CellTempAvg_C
  slr_VHAL_HVBCellVoltMax_mV : BusSelector  OutputSignals=VHAL_HVBCellVoltMax_mV
  slr_VHAL_HVBCellVoltMin_mV : BusSelector  OutputSignals=VHAL_HVBCellVoltMin_mV
  slr_VHAL_HVBMTempMax_C : BusSelector  OutputSignals=VHAL_HVBMTempMax_C
  slr_VHAL_HVBMTempMin_C : BusSelector  OutputSignals=VHAL_HVBMTempMin_C
  slr_VHAL_MaxCellTempNum_enum : BusSelector  OutputSignals=VHAL_MaxCellTempNum_enum
  slr_VHAL_MaxCellVoltNum_enum : BusSelector  OutputSignals=VHAL_MaxCellVoltNum_enum
  slr_VHAL_MinCellTempNum_enum : BusSelector  OutputSignals=VHAL_MinCellTempNum_enum
  slr_VHAL_MinCellVoltNum_enum : BusSelector  OutputSignals=VHAL_MinCellVoltNum_enum
  VINP_CellTempAvg_C : Outport
  VINP_HVBCellVoltMax_mV : Outport  Port=2
  VINP_HVBCellVoltMin_mV : Outport  Port=3
  VINP_HVBMTempMax_C : Outport  Port=4
  VINP_HVBMTempMin_C : Outport  Port=5
  VINP_MaxCellTempNum_enum : Outport  Port=6
  VINP_MaxCellVoltNum_enum : Outport  Port=7
  VINP_MinCellTempNum_enum : Outport  Port=8
  VINP_MinCellVoltNum_enum : Outport  Port=9
  wires:
  BHAL_outputs/1 -> [BHAL_outputs]
  inp_CanValid_bus/1 -> [inp_CanValid_bus]
  [BHAL_outputs] -> slr_VHAL_CellTempAvg_C/1
  slr_VHAL_CellTempAvg_C/1 -> CellTempAvg/1  "<VHAL_CellTempAvg_C>"
  True_VHAL_CellTempAvg_C/1 -> CellTempAvg/2
  [inp_CanValid_bus] -> slr1_1/1
  slr1_1/1 -> CellTempAvg/3  "<VINP_CANMsgValidBMS4_flg>"
  CellTempAvg/1 -> VINP_CellTempAvg_C/1  "VINP_CellTempAvg_C"
  CellTempAvg/2 -> Terminator_1/1
  [BHAL_outputs] -> slr_VHAL_HVBCellVoltMax_mV/1
  slr_VHAL_HVBCellVoltMax_mV/1 -> HVBCellVoltMax/1  "<VHAL_HVBCellVoltMax_mV>"
  True_VHAL_HVBCellVoltMax_mV/1 -> HVBCellVoltMax/2
  [inp_CanValid_bus] -> slr1_2/1
  slr1_2/1 -> HVBCellVoltMax/3  "<VINP_CANMsgValidBMS4_flg>"
  HVBCellVoltMax/1 -> VINP_HVBCellVoltMax_mV/1  "VINP_HVBCellVoltMax_mV"
  HVBCellVoltMax/2 -> Terminator_2/1
  [BHAL_outputs] -> slr_VHAL_HVBCellVoltMin_mV/1
  slr_VHAL_HVBCellVoltMin_mV/1 -> HVBCellVoltMin/1  "<VHAL_HVBCellVoltMin_mV>"
  True_VHAL_HVBCellVoltMin_mV/1 -> HVBCellVoltMin/2
  [inp_CanValid_bus] -> slr1_3/1
  slr1_3/1 -> HVBCellVoltMin/3  "<VINP_CANMsgValidBMS4_flg>"
  HVBCellVoltMin/1 -> VINP_HVBCellVoltMin_mV/1  "VINP_HVBCellVoltMin_mV"
  HVBCellVoltMin/2 -> Terminator_3/1
  [BHAL_outputs] -> slr_VHAL_HVBMTempMax_C/1
  slr_VHAL_HVBMTempMax_C/1 -> HVBMTempMax/1  "<VHAL_HVBMTempMax_C>"
  True_VHAL_HVBMTempMax_C/1 -> HVBMTempMax/2
  [inp_CanValid_bus] -> slr1_4/1
  slr1_4/1 -> HVBMTempMax/3  "<VINP_CANMsgValidBMS4_flg>"
  HVBMTempMax/1 -> VINP_HVBMTempMax_C/1  "VINP_HVBMTempMax_C"
  HVBMTempMax/2 -> Terminator_4/1
  [BHAL_outputs] -> slr_VHAL_HVBMTempMin_C/1
  slr_VHAL_HVBMTempMin_C/1 -> HVBMTempMin/1  "<VHAL_HVBMTempMin_C>"
  True_VHAL_HVBMTempMin_C/1 -> HVBMTempMin/2
  [inp_CanValid_bus] -> slr1_5/1
  slr1_5/1 -> HVBMTempMin/3  "<VINP_CANMsgValidBMS4_flg>"
  HVBMTempMin/1 -> VINP_HVBMTempMin_C/1  "VINP_HVBMTempMin_C"
  HVBMTempMin/2 -> Terminator_5/1
  [BHAL_outputs] -> slr_VHAL_MaxCellTempNum_enum/1
  slr_VHAL_MaxCellTempNum_enum/1 -> MaxCellTempNum/1  "<VHAL_MaxCellTempNum_enum>"
  True_VHAL_MaxCellTempNum_enum/1 -> MaxCellTempNum/2
  [inp_CanValid_bus] -> slr1_6/1
  slr1_6/1 -> MaxCellTempNum/3  "<VINP_CANMsgValidBMS4_flg>"
  MaxCellTempNum/1 -> VINP_MaxCellTempNum_enum/1  "VINP_MaxCellTempNum_enum"
  MaxCellTempNum/2 -> Terminator_6/1
  [BHAL_outputs] -> slr_VHAL_MaxCellVoltNum_enum/1
  slr_VHAL_MaxCellVoltNum_enum/1 -> MaxCellVoltNum/1  "<VHAL_MaxCellVoltNum_enum>"
  True_VHAL_MaxCellVoltNum_enum/1 -> MaxCellVoltNum/2
  [inp_CanValid_bus] -> slr1_7/1
  slr1_7/1 -> MaxCellVoltNum/3  "<VINP_CANMsgValidBMS4_flg>"
  MaxCellVoltNum/1 -> VINP_MaxCellVoltNum_enum/1  "VINP_MaxCellVoltNum_enum"
  MaxCellVoltNum/2 -> Terminator_7/1
  [BHAL_outputs] -> slr_VHAL_MinCellTempNum_enum/1
  slr_VHAL_MinCellTempNum_enum/1 -> MinCellTempNum/1  "<VHAL_MinCellTempNum_enum>"
  True_VHAL_MinCellTempNum_enum/1 -> MinCellTempNum/2
  [inp_CanValid_bus] -> slr1_8/1
  slr1_8/1 -> MinCellTempNum/3  "<VINP_CANMsgValidBMS4_flg>"
  MinCellTempNum/1 -> VINP_MinCellTempNum_enum/1  "VINP_MinCellTempNum_enum"
  MinCellTempNum/2 -> Terminator_8/1
  [BHAL_outputs] -> slr_VHAL_MinCellVoltNum_enum/1
  slr_VHAL_MinCellVoltNum_enum/1 -> MinCellVoltNum/1  "<VHAL_MinCellVoltNum_enum>"
  True_VHAL_MinCellVoltNum_enum/1 -> MinCellVoltNum/2
  [inp_CanValid_bus] -> slr1_9/1
  slr1_9/1 -> MinCellVoltNum/3  "<VINP_CANMsgValidBMS4_flg>"
  MinCellVoltNum/1 -> VINP_MinCellVoltNum_enum/1  "VINP_MinCellVoltNum_enum"
  MinCellVoltNum/2 -> Terminator_9/1

== system inp/INP/CAN3/SignalCheck/BMS5 ==
  BHAL_outputs : Inport
  inp_CanValid_bus : Inport  Port=2
  HVInVolt : FVT_lib/inp/can_signal_template  SystemSampleTime=-1  VariantActivationTime=update diagram  Latency=0  AutoFrameSizeCalculation=off
      link override defval: Value=KINP_HVInVolt_V_defval
      link override ovrdflg: Value=KINP_HVInVolt_V_ovrdflg
      link override ovrdval: Value=KINP_HVInVolt_V_ovrdval
  LVBattDet12V : FVT_lib/inp/can_signal_template  SystemSampleTime=-1  VariantActivationTime=update diagram  Latency=0  AutoFrameSizeCalculation=off
      link override defval: Value=KINP_LVBattDet12V_V_defval
      link override ovrdflg: Value=KINP_LVBattDet12V_V_ovrdflg
      link override ovrdval: Value=KINP_LVBattDet12V_V_ovrdval
  OBCACCSLimit : FVT_lib/inp/can_signal_template  SystemSampleTime=-1  VariantActivationTime=update diagram  Latency=0  AutoFrameSizeCalculation=off
      link override defval: Value=KINP_OBCACCSLimit_A_defval
      link override ovrdflg: Value=KINP_OBCACCSLimit_A_ovrdflg
      link override ovrdval: Value=KINP_OBCACCSLimit_A_ovrdval
  OBCDCCurLm : FVT_lib/inp/can_signal_template  SystemSampleTime=-1  VariantActivationTime=update diagram  Latency=0  AutoFrameSizeCalculation=off
      link override defval: Value=KINP_OBCDCCurLm_A_defval
      link override ovrdflg: Value=KINP_OBCDCCurLm_A_ovrdflg
      link override ovrdval: Value=KINP_OBCDCCurLm_A_ovrdval
  OBCDCVoltLm : FVT_lib/inp/can_signal_template  SystemSampleTime=-1  VariantActivationTime=update diagram  Latency=0  AutoFrameSizeCalculation=off
      link override defval: Value=KINP_OBCDCVoltLm_V_defval
      link override ovrdflg: Value=KINP_OBCDCVoltLm_V_ovrdflg
      link override ovrdval: Value=KINP_OBCDCVoltLm_V_ovrdval
  Terminator_{1..5} (5 alike) : Terminator
  True_VHAL_HVInVolt_V : Constant  Value=TRUE  OutDataTypeStr=boolean
  True_VHAL_LVBattDet12V_V : Constant  Value=TRUE  OutDataTypeStr=boolean
  True_VHAL_OBCACCSLimit_A : Constant  Value=TRUE  OutDataTypeStr=boolean
  True_VHAL_OBCDCCurLm_A : Constant  Value=TRUE  OutDataTypeStr=boolean
  True_VHAL_OBCDCVoltLm_V : Constant  Value=TRUE  OutDataTypeStr=boolean
  slr1_{1..5} (5 alike) : BusSelector  OutputSignals=VINP_CANMsgValidBMS5_flg
  slr_VHAL_HVInVolt_V : BusSelector  OutputSignals=VHAL_HVInVolt_V
  slr_VHAL_LVBattDet12V_V : BusSelector  OutputSignals=VHAL_LVBattDet12V_V
  slr_VHAL_OBCACCSLimit_A : BusSelector  OutputSignals=VHAL_OBCACCSLimit_A
  slr_VHAL_OBCDCCurLm_A : BusSelector  OutputSignals=VHAL_OBCDCCurLm_A
  slr_VHAL_OBCDCVoltLm_V : BusSelector  OutputSignals=VHAL_OBCDCVoltLm_V
  VINP_HVInVolt_V : Outport
  VINP_LVBattDet12V_V : Outport  Port=2
  VINP_OBCACCSLimit_A : Outport  Port=3
  VINP_OBCDCCurLm_A : Outport  Port=4
  VINP_OBCDCVoltLm_V : Outport  Port=5
  wires:
  BHAL_outputs/1 -> [BHAL_outputs]
  inp_CanValid_bus/1 -> [inp_CanValid_bus]
  [BHAL_outputs] -> slr_VHAL_HVInVolt_V/1
  slr_VHAL_HVInVolt_V/1 -> HVInVolt/1  "<VHAL_HVInVolt_V>"
  True_VHAL_HVInVolt_V/1 -> HVInVolt/2
  [inp_CanValid_bus] -> slr1_1/1
  slr1_1/1 -> HVInVolt/3  "<VINP_CANMsgValidBMS5_flg>"
  HVInVolt/1 -> VINP_HVInVolt_V/1  "VINP_HVInVolt_V"
  HVInVolt/2 -> Terminator_1/1
  [BHAL_outputs] -> slr_VHAL_LVBattDet12V_V/1
  slr_VHAL_LVBattDet12V_V/1 -> LVBattDet12V/1  "<VHAL_LVBattDet12V_V>"
  True_VHAL_LVBattDet12V_V/1 -> LVBattDet12V/2
  [inp_CanValid_bus] -> slr1_2/1
  slr1_2/1 -> LVBattDet12V/3  "<VINP_CANMsgValidBMS5_flg>"
  LVBattDet12V/1 -> VINP_LVBattDet12V_V/1  "VINP_LVBattDet12V_V"
  LVBattDet12V/2 -> Terminator_2/1
  [BHAL_outputs] -> slr_VHAL_OBCACCSLimit_A/1
  slr_VHAL_OBCACCSLimit_A/1 -> OBCACCSLimit/1  "<VHAL_OBCACCSLimit_A>"
  True_VHAL_OBCACCSLimit_A/1 -> OBCACCSLimit/2
  [inp_CanValid_bus] -> slr1_3/1
  slr1_3/1 -> OBCACCSLimit/3  "<VINP_CANMsgValidBMS5_flg>"
  OBCACCSLimit/1 -> VINP_OBCACCSLimit_A/1  "VINP_OBCACCSLimit_A"
  OBCACCSLimit/2 -> Terminator_3/1
  [BHAL_outputs] -> slr_VHAL_OBCDCCurLm_A/1
  slr_VHAL_OBCDCCurLm_A/1 -> OBCDCCurLm/1  "<VHAL_OBCDCCurLm_A>"
  True_VHAL_OBCDCCurLm_A/1 -> OBCDCCurLm/2
  [inp_CanValid_bus] -> slr1_4/1
  slr1_4/1 -> OBCDCCurLm/3  "<VINP_CANMsgValidBMS5_flg>"
  OBCDCCurLm/1 -> VINP_OBCDCCurLm_A/1  "VINP_OBCDCCurLm_A"
  OBCDCCurLm/2 -> Terminator_4/1
  [BHAL_outputs] -> slr_VHAL_OBCDCVoltLm_V/1
  slr_VHAL_OBCDCVoltLm_V/1 -> OBCDCVoltLm/1  "<VHAL_OBCDCVoltLm_V>"
  True_VHAL_OBCDCVoltLm_V/1 -> OBCDCVoltLm/2
  [inp_CanValid_bus] -> slr1_5/1
  slr1_5/1 -> OBCDCVoltLm/3  "<VINP_CANMsgValidBMS5_flg>"
  OBCDCVoltLm/1 -> VINP_OBCDCVoltLm_V/1  "VINP_OBCDCVoltLm_V"
  OBCDCVoltLm/2 -> Terminator_5/1
